simulink model "Simulink_Program_June30_K2andK3"  (R2023b)
settings: Solver=VariableStepAuto  StartTime=0.0  StopTime=1  RelTol=1e-3
libraries: fl_lib x11, nesl_utility x9, ee_lib x7, SignalEditorBlockLib x1
settings Model: Creator=romul  LastModifiedBy=OWNER

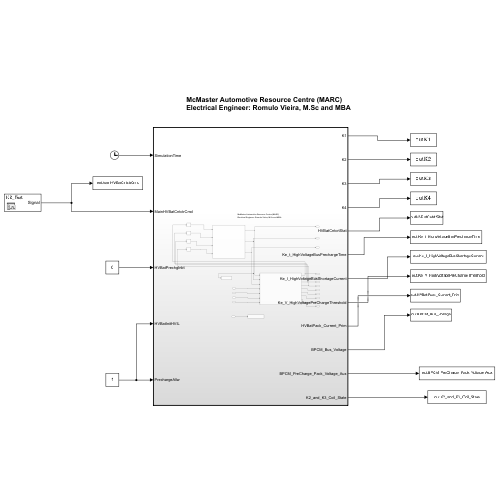
[thumbnail: Simulink's stored preview of the top-level diagram]
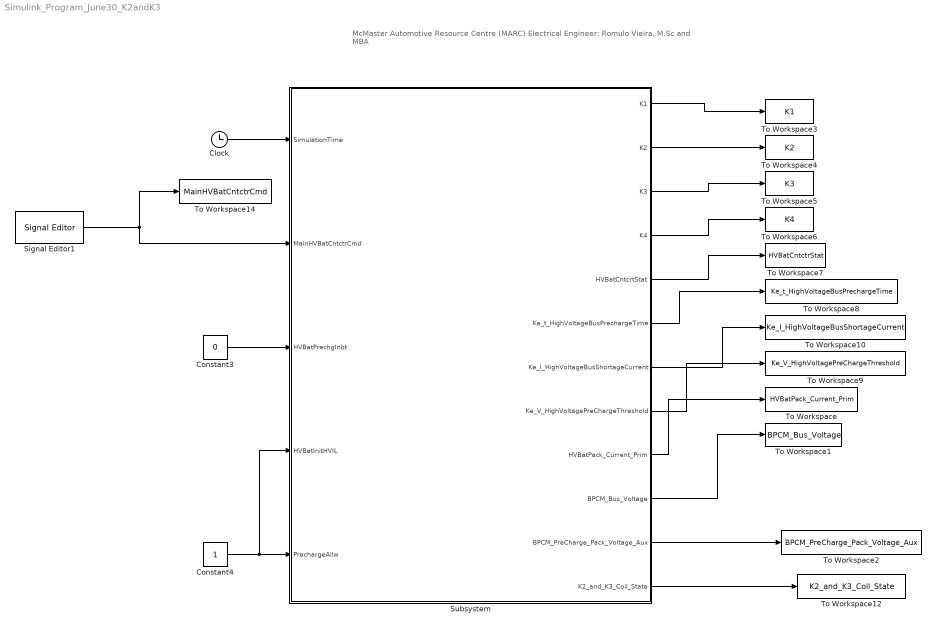
== system Simulink_Program_June30_K2andK3 ==
  note: McMaster Automotive Resource Centre (MARC)
      | Electrical Engineer: Romulo Vieira, M.Sc and MBA
  Clock : Clock
  Constant3 : Constant  Value=0
  Constant4 : Constant
  Signal Editor1 : SignalEditorBlockLib/Signal Editor  FileName=K2_Test.mat  ActiveScenario=K2_Test  ActiveSignal=Signal  IsBus=off  OutputBusObjectStr=Bus: BusObject  SampleTime=0  Interpolate=off  ZeroCross=off  OutputAfterFinalValue=Setting to zero  Unit=inherit  PreserveSignalName=on  ApplySigPropsToAllScenarios=on  ApplySigPropsToAllSignals=off
  Subsystem : Subsystem  TreatAsAtomicUnit=on
  To Workspace : ToWorkspace  VariableName=HVBatPack_Current_Prim  SampleTime=-1
  To Workspace1 : ToWorkspace  VariableName=BPCM_Bus_Voltage  SampleTime=-1
  To Workspace10 : ToWorkspace  VariableName=Ke_I_HighVoltageBusShortageCurrent  SampleTime=-1
  To Workspace12 : ToWorkspace  VariableName=K2_and_K3_Coil_State  SampleTime=-1
  To Workspace14 : ToWorkspace  VariableName=MainHVBatCntctrCmd  SaveFormat=Timeseries  SampleTime=-1
  To Workspace2 : ToWorkspace  VariableName=BPCM_PreCharge_Pack_Voltage_Aux  SampleTime=-1
  To Workspace3 : ToWorkspace  VariableName=K1  SaveFormat=Timeseries  SampleTime=-1
  To Workspace4 : ToWorkspace  VariableName=K2  SaveFormat=Timeseries  SampleTime=-1
  To Workspace5 : ToWorkspace  VariableName=K3  SaveFormat=Timeseries  SampleTime=-1
  To Workspace6 : ToWorkspace  VariableName=K4  SampleTime=-1
  To Workspace7 : ToWorkspace  VariableName=HVBatCntctrStat  SampleTime=-1
  To Workspace8 : ToWorkspace  VariableName=Ke_t_HighVoltageBusPrechargeTime  SampleTime=-1
  To Workspace9 : ToWorkspace  VariableName=Ke_V_HighVoltagePreChargeThreshold  SampleTime=-1
  wires:
  Subsystem/4(K4) -> To Workspace6/1
  Subsystem/12(K2_and_K3_Coil_State) -> To Workspace12/1
  Subsystem/7(Ke_I_HighVoltageBusShortageCurrent) -> To Workspace10/1
  Subsystem/1(K1) -> To Workspace3/1
  Clock/1 -> Subsystem/1(SimulationTime)
  Constant3/1 -> Subsystem/3(HVBatPrechgInbt)
  Subsystem/2(K2) -> To Workspace4/1
  Subsystem/8(Ke_V_HighVoltagePreChargeThreshold) -> To Workspace9/1
  Subsystem/3(K3) -> To Workspace5/1
  Constant4/1 -> Subsystem/5(PrechargeAllw), Subsystem/4(HVBatInitHVIL)
  Subsystem/11(BPCM_PreCharge_Pack_Voltage_Aux) -> To Workspace2/1
  Subsystem/6(Ke_t_HighVoltageBusPrechargeTime) -> To Workspace8/1
  Subsystem/5(HVBatCntcrtStat) -> To Workspace7/1
  Subsystem/10(BPCM_Bus_Voltage) -> To Workspace1/1
  Subsystem/9(HVBatPack_Current_Prim) -> To Workspace/1
  Signal Editor1/1 -> To Workspace14/1, Subsystem/2(MainHVBatCntctrCmd)

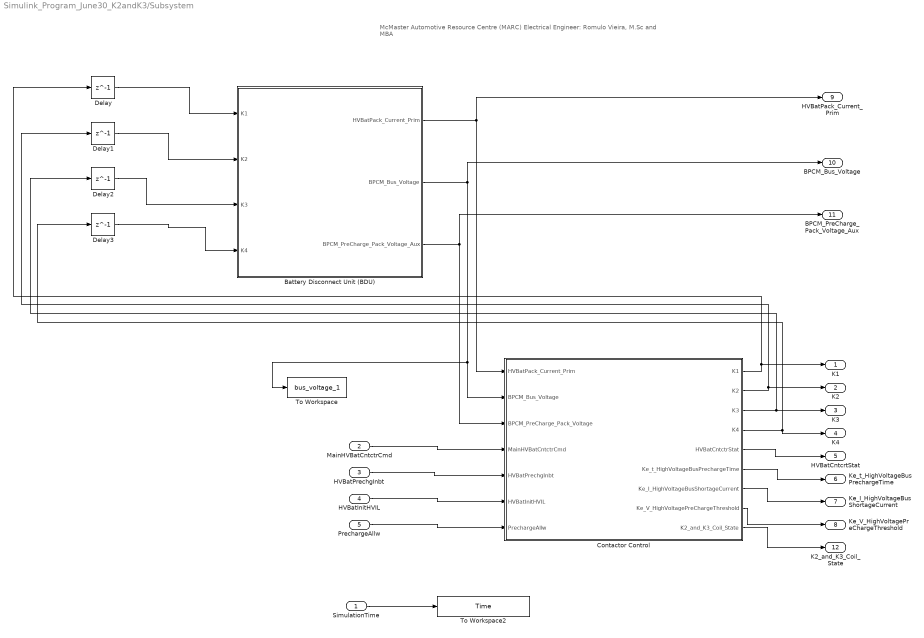
== system Simulink_Program_June30_K2andK3/Subsystem ==
  note: McMaster Automotive Resource Centre (MARC)
      | Electrical Engineer: Romulo Vieira, M.Sc and MBA
  SimulationTime : Inport
  MainHVBatCntctrCmd : Inport  Port=2
  HVBatPrechgInbt : Inport  Port=3
  HVBatInitHVIL : Inport  Port=4
  PrechargeAllw : Inport  Port=5
  Battery Disconnect Unit (BDU) : Subsystem  TreatAsAtomicUnit=on
  Contactor Control : Subsystem  TreatAsAtomicUnit=on
  Delay{,1..3} (4 alike) : Delay  DelayLength=1
  To Workspace : ToWorkspace  VariableName=bus_voltage_1  SaveFormat=Timeseries  SampleTime=-1
  To Workspace2 : ToWorkspace  VariableName=Time  SampleTime=0.001
  K1 : Outport
  K2 : Outport  Port=2
  K3 : Outport  Port=3
  K4 : Outport  Port=4
  HVBatCntcrtStat : Outport  Port=5
  Ke_t_HighVoltageBusPrechargeTime : Outport  Port=6
  Ke_I_HighVoltageBusShortageCurrent : Outport  Port=7
  Ke_V_HighVoltagePreChargeThreshold : Outport  Port=8
  HVBatPack_Current_Prim : Outport  Port=9
  BPCM_Bus_Voltage : Outport  Port=10
  BPCM_PreCharge_Pack_Voltage_Aux : Outport  Port=11
  K2_and_K3_Coil_State : Outport  Port=12
  wires:
  Battery Disconnect Unit (BDU)/1(HVBatPack_Current_Prim) -> HVBatPack_Current_Prim/1, Contactor Control/1(HVBatPack_Current_Prim)
  HVBatPrechgInbt/1 -> Contactor Control/5(HVBatPrechgInbt)
  HVBatInitHVIL/1 -> Contactor Control/6(HVBatInitHVIL)
  PrechargeAllw/1 -> Contactor Control/7(PrechargeAllw)
  Contactor Control/1(K1) -> K1/1, Delay/1
  Contactor Control/2(K2) -> Delay1/1, K2/1
  Contactor Control/3(K3) -> Delay2/1, K3/1
  Contactor Control/4(K4) -> Delay3/1, K4/1
  Contactor Control/5(HVBatCntctrStat) -> HVBatCntcrtStat/1
  Contactor Control/6(Ke_t_HighVoltageBusPrechargeTime) -> Ke_t_HighVoltageBusPrechargeTime/1
  Contactor Control/7(Ke_I_HighVoltageBusShortageCurrent) -> Ke_I_HighVoltageBusShortageCurrent/1
  Contactor Control/8(Ke_V_HighVoltagePreChargeThreshold) -> Ke_V_HighVoltagePreChargeThreshold/1
  Battery Disconnect Unit (BDU)/3(BPCM_PreCharge_Pack_Voltage_Aux) -> BPCM_PreCharge_Pack_Voltage_Aux/1, Contactor Control/3(BPCM_PreCharge_Pack_Voltage)
  Delay/1 -> Battery Disconnect Unit (BDU)/1(K1)
  Delay1/1 -> Battery Disconnect Unit (BDU)/2(K2)
  Delay2/1 -> Battery Disconnect Unit (BDU)/3(K3)
  Delay3/1 -> Battery Disconnect Unit (BDU)/4(K4)
  SimulationTime/1 -> To Workspace2/1
  Battery Disconnect Unit (BDU)/2(BPCM_Bus_Voltage) -> BPCM_Bus_Voltage/1, Contactor Control/2(BPCM_Bus_Voltage), To Workspace/1
  Contactor Control/9(K2_and_K3_Coil_State) -> K2_and_K3_Coil_State/1
  MainHVBatCntctrCmd/1 -> Contactor Control/4(MainHVBatCntctrCmd)

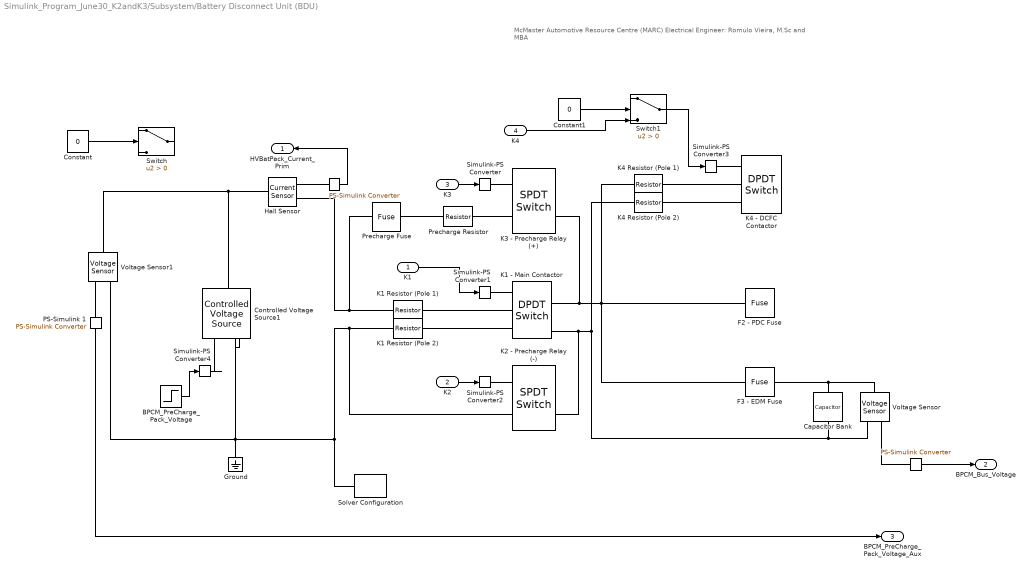
== system Simulink_Program_June30_K2andK3/Subsystem/Battery Disconnect Unit (BDU) ==
  note: McMaster Automotive Resource Centre (MARC)
      | Electrical Engineer: Romulo Vieira, M.Sc and MBA
  K1 : Inport
  K2 : Inport  Port=2
  K3 : Inport  Port=3
  K4 : Inport  Port=4
  "   " : nesl_utility/PS-Simulink Converter  PhysicalDomain=network_engine_domain  SubClassName=ps_output  LeftPortType=input  RightPortType=output  PseudoPeriodic=off  Frequencies=[]  VectorFormat=inherit  Unit=inherit  AffineConversion=off
  " " : nesl_utility/PS-Simulink Converter  PhysicalDomain=network_engine_domain  SubClassName=ps_output  LeftPortType=input  RightPortType=output  PseudoPeriodic=off  Frequencies=[]  VectorFormat=inherit  Unit=inherit  AffineConversion=off
  BPCM_PreCharge_Pack_Voltage : Step  Time=0  After=450  SampleTime=0.001
  Capacitor Bank : fl_lib/Electrical/Electrical Elements/Capacitor  c=750e-6 F  r=1e-6 Ohm  g=0 1/Ohm  i_specify=off  i_priority=None  i=0 A  i_nominal_specify=off  i_nominal_unit=A  i_nominal_value=1  v_specify=off  v_priority=None  v=0 V  v_nominal_specify=off  v_nominal_unit=V  v_nominal_value=1  vc_specify=on  vc_priority=High  vc=0 V  vc_nominal_specify=off  vc_nominal_unit=V  vc_nominal_value=1
  Constant : Constant  Value=0
  Constant1 : Constant  Value=0
  Controlled Voltage Source1 : fl_lib/Electrical/Electrical Sources/Controlled Voltage Source
  F2 - PDC Fuse : ee_lib/Switches & Breakers/Fuse  prm=1  I_rated=125 A  melt_margin=1  T_fuse=0 s  I2t=1 A^2*s  I_vec=[1.9, 2, 2.5, 30] A  t_vec=[10000, 1, .3, .001] s  R_closed=0.01 Ohm  G_open=1e-8 1/Ohm  exposemeasurement=ee.enum.exposemeasurement.hidden
      settings: InternalSimscapePortConfiguration="{\"Bottom\":[],\"Left\":[{\"id\":\"p\",\"label\":\"\",\"type\":\"foundation.electrical.electrical\"}],\"Right\":[{\"id\":\"n\",\"label\":\"\",\"type\":\"foundation.electrical.electrical\"}],\"Top\":[]}"
  F3 - EDM Fuse : ee_lib/Switches & Breakers/Fuse  prm=1  I_rated=600 A  melt_margin=1  T_fuse=0 s  I2t=1 A^2*s  I_vec=[1.9, 2, 2.5, 30] A  t_vec=[10000, 1, .3, .001] s  R_closed=0.01 Ohm  G_open=1e-8 1/Ohm  exposemeasurement=ee.enum.exposemeasurement.hidden
      settings: InternalSimscapePortConfiguration="{\"Bottom\":[],\"Left\":[{\"id\":\"p\",\"label\":\"\",\"type\":\"foundation.electrical.electrical\"}],\"Right\":[{\"id\":\"n\",\"label\":\"\",\"type\":\"foundation.electrical.electrical\"}],\"Top\":[]}"
  Ground : fl_lib/Electrical/Electrical Elements/Electrical Reference
  Hall Sensor : fl_lib/Electrical/Electrical Sensors/Current Sensor
  K1 - Main Contactor : ee_lib/Switches & Breakers/DPDT Switch  R_closed=0.01 Ohm  G_open=1e-6 S  Threshold=0.5 V  Width=0 V  model_dynamics=0  t_on=1e-3 s  t_off=1e-3 s  initial_vT=0 V
      settings: InternalSimscapePortConfiguration="{\"Bottom\":[],\"Left\":[{\"id\":\"vT\",\"label\":\"vT\",\"type\":\"input\"},{\"id\":\"p1\",\"label\":\"\",\"type\":\"foundation.electrical.electrical\"},{\"id\":\"p2\",\"label\":\"\",\"type\":\"foundation.electrical.electrical\"}],\"Right\":[{\"id\":\"n11\",\"label\":\"\",\"type\":\"foundation.electrical.electrical\"},{\"id\":\"n12\",\"label\":\"\",\"type\":\"foundation.electrical.electrical\"},{\"id\":\"n21\",\"label\":\"\",\"type\":\"foundation.electrical.electrical\"},{\"id\":\"n22\",\"label\":\"\",\"type\":\"foundation.electrical.electrical\"}],\"Top\":[]}"
  K1 Resistor (Pole 1) : fl_lib/Electrical/Electrical Elements/Resistor  R=0.0003 Ohm  i_specify=off  i_priority=None  i=0 A  i_nominal_specify=off  i_nominal_unit=A  i_nominal_value=1  v_specify=off  v_priority=None  v=0 V  v_nominal_specify=off  v_nominal_unit=V  v_nominal_value=1
  K1 Resistor (Pole 2) : fl_lib/Electrical/Electrical Elements/Resistor  R=0.0003 Ohm  i_specify=off  i_priority=None  i=0 A  i_nominal_specify=off  i_nominal_unit=A  i_nominal_value=1  v_specify=off  v_priority=None  v=0 V  v_nominal_specify=off  v_nominal_unit=V  v_nominal_value=1
  K2 - Precharge Relay (-) : ee_lib/Switches & Breakers/SPDT Switch  R_closed=0.01 Ohm  G_open=1e-6 S  Threshold=0.5 V  Width=0 V  model_dynamics=0  t_on=1e-3 s  t_off=1e-3 s  initial_vT=0 V
  K3 - Precharge Relay (+) : ee_lib/Switches & Breakers/SPDT Switch  R_closed=0.01 Ohm  G_open=1e-6 S  Threshold=0.5 V  Width=0 V  model_dynamics=0  t_on=1e-3 s  t_off=1e-3 s  initial_vT=0 V
  K4 - DCFC Contactor : ee_lib/Switches & Breakers/DPDT Switch  R_closed=0.01 Ohm  G_open=1e-6 S  Threshold=0.5 V  Width=0 V  model_dynamics=0  t_on=1e-3 s  t_off=1e-3 s  initial_vT=0 V
      settings: InternalSimscapePortConfiguration="{\"Bottom\":[],\"Left\":[{\"id\":\"vT\",\"label\":\"vT\",\"type\":\"input\"},{\"id\":\"p1\",\"label\":\"\",\"type\":\"foundation.electrical.electrical\"},{\"id\":\"p2\",\"label\":\"\",\"type\":\"foundation.electrical.electrical\"}],\"Right\":[{\"id\":\"n11\",\"label\":\"\",\"type\":\"foundation.electrical.electrical\"},{\"id\":\"n12\",\"label\":\"\",\"type\":\"foundation.electrical.electrical\"},{\"id\":\"n21\",\"label\":\"\",\"type\":\"foundation.electrical.electrical\"},{\"id\":\"n22\",\"label\":\"\",\"type\":\"foundation.electrical.electrical\"}],\"Top\":[]}"
  K4 Resistor (Pole 1) : fl_lib/Electrical/Electrical Elements/Resistor  R=0.0003 Ohm  i_specify=off  i_priority=None  i=0 A  i_nominal_specify=off  i_nominal_unit=A  i_nominal_value=1  v_specify=off  v_priority=None  v=0 V  v_nominal_specify=off  v_nominal_unit=V  v_nominal_value=1
  K4 Resistor (Pole 2) : fl_lib/Electrical/Electrical Elements/Resistor  R=0.0003 Ohm  i_specify=off  i_priority=None  i=0 A  i_nominal_specify=off  i_nominal_unit=A  i_nominal_value=1  v_specify=off  v_priority=None  v=0 V  v_nominal_specify=off  v_nominal_unit=V  v_nominal_value=1
  PS-Simulink 1 : nesl_utility/PS-Simulink Converter  PhysicalDomain=network_engine_domain  SubClassName=ps_output  LeftPortType=input  RightPortType=output  PseudoPeriodic=off  Frequencies=[]  VectorFormat=inherit  Unit=inherit  AffineConversion=off
  Precharge Fuse : ee_lib/Switches & Breakers/Fuse  prm=1  I_rated=600 A  melt_margin=1  T_fuse=0 s  I2t=1 A^2*s  I_vec=[1.9, 2, 2.5, 30] A  t_vec=[10000, 1, .3, .001] s  R_closed=0.01 Ohm  G_open=1e-8 1/Ohm  exposemeasurement=ee.enum.exposemeasurement.hidden
      settings: InternalSimscapePortConfiguration="{\"Bottom\":[],\"Left\":[{\"id\":\"p\",\"label\":\"\",\"type\":\"foundation.electrical.electrical\"}],\"Right\":[{\"id\":\"n\",\"label\":\"\",\"type\":\"foundation.electrical.electrical\"}],\"Top\":[]}"
  Precharge Resistor : fl_lib/Electrical/Electrical Elements/Resistor  R=25 Ohm  i_specify=off  i_priority=None  i=0 A  i_nominal_specify=off  i_nominal_unit=A  i_nominal_value=1  v_specify=off  v_priority=None  v=0 V  v_nominal_specify=off  v_nominal_unit=V  v_nominal_value=1
  Simulink-PS Converter{,1..3} (4 alike) : nesl_utility/Simulink-PS Converter  PhysicalDomain=network_engine_domain  SubClassName=ps_input  LeftPortType=input  RightPortType=output  PseudoPeriodic=off  Frequencies=[]  NoiseDistribution=none  NoiseParameters=[]  Unit=1  AffineConversion=off  FilteringAndDerivatives=provide  SimscapeFilterOrder=1  InputFilterTimeConstant=0.001  UdotUserProvided=0
  Simulink-PS Converter4 : nesl_utility/Simulink-PS Converter  PhysicalDomain=network_engine_domain  SubClassName=ps_input  LeftPortType=input  RightPortType=output  PseudoPeriodic=off  Frequencies=[]  NoiseDistribution=none  NoiseParameters=[]  Unit=1  AffineConversion=off  FilteringAndDerivatives=filter  SimscapeFilterOrder=1  InputFilterTimeConstant=0.0000001  UdotUserProvided=0
  Solver Configuration : nesl_utility/Solver Configuration  PhysicalDomain=network_engine_domain  SubClassName=solver  LeftPortType=input  RightPortType=generic  Tones=[]  Harmonics=[]  SimulateNoise=off  Profile=off  UseLocalSampling=off  EnableSwitchedLinearOptims=on  FrequencyDomain=off  UseCCode=off  RelTol=0.001  AbsTol=0.001  MinStep=1e-09  ToWorkspace=off  RevertToSquareIcSolve=off  NumHomotopyIterations=100  PhasorMode=off  PhasorModeNumHarmonics=1  ConsistencySolver=NEWTON_XTOL_AFTER_FTOL  IndexReductionMethod=DerivativeReplacement  DoDC=off  ResidualTolerance=1e-09  ConsistencyTolSource=GLOBAL  ConsistencyAbsTol=0.001  ConsistencyRelTol=0.001  ConsistencyTolFactor=0.001  UseLocalSolver=off  LocalSolverChoice=NE_BACKWARD_EULER_ADVANCER  ResolveIndetEquations=on  FunctionEvalNumThread=1  LocalSolverSampleTime=0.001  DoFixedCost=off  MaxNonlinIter=3  MaxModeIter=2  ComputeImpulses=off  ImpulseIterations=2  LinearAlgebra=auto  LinearAlgebraNumThread=0  EquationFormulation=NE_TIME_EF  DelaysMemoryBudget=1024  AutomaticFiltering=on  FilteringTimeConstant=0.001  PartitionStorageMethod=AS_NEEDED  PartitionMemoryBudget=1024  PartitionMethod=ROBUST  MultibodyUseLocalSolver=off  MultibodyLocalSolverChoice=ODE1  MultibodyLocalSolverSampleTime=0.001
  Switch : Switch  Criteria=u2 > Threshold  SaturateOnIntegerOverflow=off  InputSameDT=off
  Switch1 : Switch  Criteria=u2 > Threshold  SaturateOnIntegerOverflow=off  InputSameDT=off
  Voltage Sensor : fl_lib/Electrical/Electrical Sensors/Voltage Sensor
  Voltage Sensor1 : fl_lib/Electrical/Electrical Sensors/Voltage Sensor
  HVBatPack_Current_Prim : Outport
  BPCM_Bus_Voltage : Outport  Port=2
  BPCM_PreCharge_Pack_Voltage_Aux : Outport  Port=3
  wires:
  Switch1/1 -> Simulink-PS Converter3/1
  K3/1 -> Simulink-PS Converter/1
  "   "/1 -> HVBatPack_Current_Prim/1
  K2/1 -> Simulink-PS Converter2/1
  BPCM_PreCharge_Pack_Voltage/1 -> Simulink-PS Converter4/1
  PS-Simulink 1/1 -> BPCM_PreCharge_Pack_Voltage_Aux/1
  " "/1 -> BPCM_Bus_Voltage/1
  K1/1 -> Simulink-PS Converter1/1
  Constant1/1 -> Switch1/2
  K4/1 -> Switch1/3
  ? -> Switch1/1
  ? -> Switch/1
  ? -> Switch/3
  Constant/1 -> Switch/2
  connections:
  K1 Resistor (Pole 2)/LConn1 -- K1 - Main Contactor/LConn3
  Capacitor Bank/LConn1 -- Voltage Sensor/LConn1 -- F3 - EDM Fuse/LConn1
  K2 - Precharge Relay (-)/RConn2 -- K1 - Main Contactor/RConn4 -- Voltage Sensor/RConn2 -- Capacitor Bank/RConn1 -- K4 Resistor (Pole 2)/RConn1
  Hall Sensor/RConn2 -- Precharge Fuse/LConn1 -- K1 Resistor (Pole 1)/RConn1
  K3 - Precharge Relay (+)/RConn2 -- K4 Resistor (Pole 1)/RConn1 -- F2 - PDC Fuse/RConn1 -- F3 - EDM Fuse/RConn1 -- K1 - Main Contactor/RConn2
  Precharge Resistor/LConn1 -- K3 - Precharge Relay (+)/LConn2
  Simulink-PS Converter2/RConn1 -- K2 - Precharge Relay (-)/LConn1
  Precharge Resistor/RConn1 -- Precharge Fuse/RConn1
  Simulink-PS Converter1/RConn1 -- K1 - Main Contactor/LConn1
  Controlled Voltage Source1/LConn1 -- Hall Sensor/LConn1 -- Voltage Sensor1/LConn1
  Simulink-PS Converter/RConn1 -- K3 - Precharge Relay (+)/LConn1
  Voltage Sensor/RConn1 -- " "/LConn1
  K4 - DCFC Contactor/LConn1 -- Simulink-PS Converter3/RConn1
  "   "/LConn1 -- Hall Sensor/RConn1
  Simulink-PS Converter4/RConn1 -- Controlled Voltage Source1/RConn1
  Voltage Sensor1/RConn1 -- PS-Simulink 1/LConn1
  K1 Resistor (Pole 1)/LConn1 -- K1 - Main Contactor/LConn2
  Solver Configuration/RConn1 -- Ground/LConn1 -- Voltage Sensor1/RConn2 -- Controlled Voltage Source1/RConn2 -- K2 - Precharge Relay (-)/LConn2 -- K1 Resistor (Pole 2)/RConn1
  K4 - DCFC Contactor/LConn2 -- K4 Resistor (Pole 1)/LConn1
  K4 Resistor (Pole 2)/LConn1 -- K4 - DCFC Contactor/LConn3

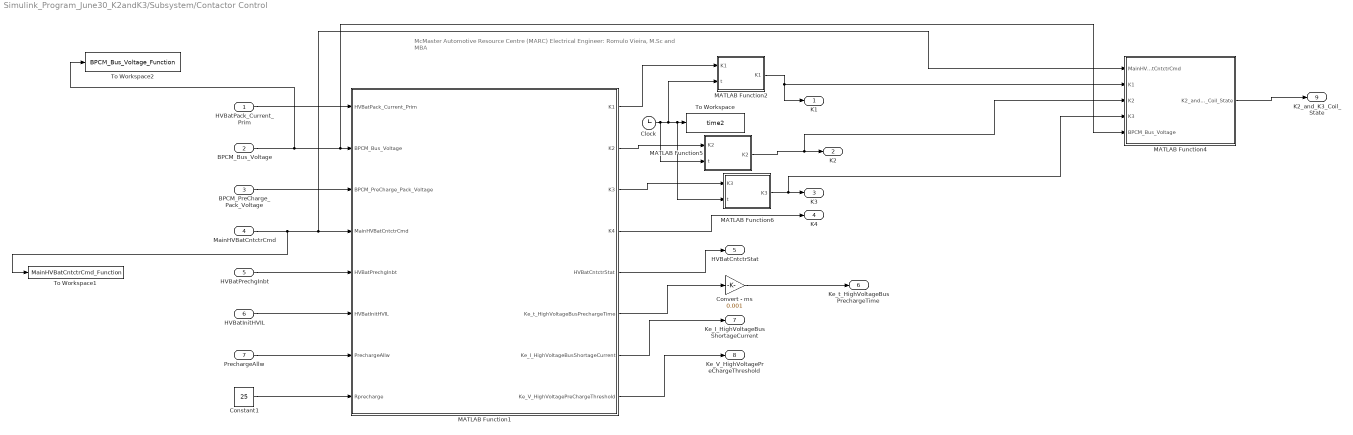
== system Simulink_Program_June30_K2andK3/Subsystem/Contactor Control ==
  note: McMaster Automotive Resource Centre (MARC)
      | Electrical Engineer: Romulo Vieira, M.Sc and MBA
  HVBatPack_Current_Prim : Inport
  BPCM_Bus_Voltage : Inport  Port=2
  BPCM_PreCharge_Pack_Voltage : Inport  Port=3
  MainHVBatCntctrCmd : Inport  Port=4
  HVBatPrechgInbt : Inport  Port=5
  HVBatInitHVIL : Inport  Port=6
  PrechargeAllw : Inport  Port=7
  Clock : Clock
  Constant1 : Constant  Value=25
  Convert - ms : Gain  Gain=0.001
  MATLAB Function1 : MATLAB Function  SystemSampleTime=0.001
  MATLAB Function2 : MATLAB Function  TreatAsAtomicUnit=on
  MATLAB Function4 : MATLAB Function  TreatAsAtomicUnit=on
  MATLAB Function5 : MATLAB Function  TreatAsAtomicUnit=on
  MATLAB Function6 : MATLAB Function  TreatAsAtomicUnit=on
  To Workspace : ToWorkspace  VariableName=time2  SampleTime=-1
  To Workspace1 : ToWorkspace  VariableName=MainHVBatCntctrCmd_Function  SaveFormat=Timeseries  SampleTime=-1
  To Workspace2 : ToWorkspace  VariableName=BPCM_Bus_Voltage_Function  SaveFormat=Timeseries  SampleTime=-1
  K1 : Outport
  K2 : Outport  Port=2
  K3 : Outport  Port=3
  K4 : Outport  Port=4
  HVBatCntctrStat : Outport  Port=5
  Ke_t_HighVoltageBusPrechargeTime : Outport  Port=6
  Ke_I_HighVoltageBusShortageCurrent : Outport  Port=7
  Ke_V_HighVoltagePreChargeThreshold : Outport  Port=8
  K2_and_K3_Coil_State : Outport  Port=9
  wires:
  HVBatPack_Current_Prim/1 -> MATLAB Function1/1(HVBatPack_Current_Prim)
  PrechargeAllw/1 -> MATLAB Function1/7(PrechargeAllw)
  BPCM_PreCharge_Pack_Voltage/1 -> MATLAB Function1/3(BPCM_PreCharge_Pack_Voltage)
  Constant1/1 -> MATLAB Function1/8(Rprecharge)
  MATLAB Function1/7(Ke_I_HighVoltageBusShortageCurrent) -> Ke_I_HighVoltageBusShortageCurrent/1
  HVBatInitHVIL/1 -> MATLAB Function1/6(HVBatInitHVIL)
  HVBatPrechgInbt/1 -> MATLAB Function1/5(HVBatPrechgInbt)
  MATLAB Function1/5(HVBatCntctrStat) -> HVBatCntctrStat/1
  MATLAB Function1/6(Ke_t_HighVoltageBusPrechargeTime) -> Convert - ms/1
  MATLAB Function1/8(Ke_V_HighVoltagePreChargeThreshold) -> Ke_V_HighVoltagePreChargeThreshold/1
  Convert - ms/1 -> Ke_t_HighVoltageBusPrechargeTime/1
  MATLAB Function4/1(K2_and_K3_Coil_State) -> K2_and_K3_Coil_State/1
  MATLAB Function1/4(K4) -> K4/1
  Clock/1 -> MATLAB Function5/2(t), MATLAB Function2/2(t), MATLAB Function6/2(t), To Workspace/1
  BPCM_Bus_Voltage/1 -> MATLAB Function4/5(BPCM_Bus_Voltage), MATLAB Function1/2(BPCM_Bus_Voltage), To Workspace2/1
  MainHVBatCntctrCmd/1 -> To Workspace1/1, MATLAB Function4/1(MainHVBatCntctrCmd), MATLAB Function1/4(MainHVBatCntctrCmd)
  MATLAB Function1/2(K2) -> MATLAB Function5/1("K2 ")
  MATLAB Function5/1(K2) -> MATLAB Function4/3(K2), K2/1
  MATLAB Function1/3(K3) -> MATLAB Function6/1("K3 ")
  MATLAB Function6/1(K3) -> MATLAB Function4/4(K3), K3/1
  MATLAB Function1/1(K1) -> MATLAB Function2/1("K1 ")
  MATLAB Function2/1(K1) -> MATLAB Function4/2(K1), K1/1

== matlab function Simulink_Program_June30_K2andK3/Subsystem/Contactor Control/MATLAB Function1 ==
  settings: updateMethod=DISCRETE
  data: HVBatPack_Current_Prim input; BPCM_Bus_Voltage input; BPCM_PreCharge_Pack_Voltage input; MainHVBatCntctrCmd input; K1 output; HVBatPrechgInbt input; HVBatInitHVIL input; PrechargeAllw input; K2 output; K3 output; K4 output; HVBatCntctrStat output; Ke_t_HighVoltageBusPrechargeTime output; Ke_I_HighVoltageBusShortageCurrent output; Ke_V_HighVoltagePreChargeThreshold output; Rprecharge input
% McMaster Automotive Resource Centre (MARC)
% Electrical Engineer: Romulo Vieira, M.Sc and MBA - PhD Candidate
function [K1, K2, K3, K4, HVBatCntctrStat, Ke_t_HighVoltageBusPrechargeTime, Ke_I_HighVoltageBusShortageCurrent, Ke_V_HighVoltagePreChargeThreshold] = prechargeSequencerNoClock( ...
     HVBatPack_Current_Prim, BPCM_Bus_Voltage, BPCM_PreCharge_Pack_Voltage, MainHVBatCntctrCmd, HVBatPrechgInbt, HVBatInitHVIL, PrechargeAllw, Rprecharge)

%-----------------------------------------------------------
% Purpose: Manage precharge relay and contactor sequence without an external clock
% Controls how the HV bus charges up safely to near pack voltage
% Tracks time window where precharge relays were active
%-----------------------------------------------------------

% Declare persistent variables (retain values across function calls)
persistent I_buffer V_buffer idx Stage HVBatCntctrStat_Aux Ke_idx fill_count last_PrechargeAllw stage2_count TimeSincePrechargeStart

% Declare constants
Buffer_length                      = 100; % Buffer to store 100 ms worth of data (1 ms sample rate in Matlab function)
Ke_V_HighVoltagePreChargeThreshold = 0.99 * BPCM_PreCharge_Pack_Voltage; % Target voltage: 98.5% of pack voltage
Unset_Ke_idx                       = -1; % Marker to indicate target not reached yet
Min_Stage2_Samples                 = 1; % Minimum time (samples) to stay in Stage 2

% Initialize persistent variables on first call
if isempty(I_buffer)
    I_buffer            = zeros(Buffer_length,1); % Precharge current buffer
    V_buffer            = zeros(Buffer_length,1); % Precharge voltage buffer
    idx                 = 1; % Index for buffers
    Stage               = 0; % Initial internal stage
    HVBatCntctrStat_Aux = 0; % Initial stage for the contactor control
    Ke_idx              = Unset_Ke_idx; % Target voltage not reached yet
    fill_count          = 0; % Counter for Stage 1 samples
    last_PrechargeAllw  = 0; % Track previous PrechargeAllw
    stage2_count        = 0; % Counter for Stage 2 duration
end

if isempty(TimeSincePrechargeStart)
    TimeSincePrechargeStart = 0;
end

% Default outputs
K1 = 0; K2 = 0; K3 = 0; K4 = 0;
HVBatCntctrStat = HVBatCntctrStat_Aux;

switch Stage
    case 0
        % All contactors off
        if MainHVBatCntctrCmd == 1 && HVBatPrechgInbt == 0 && HVBatInitHVIL == 1 && PrechargeAllw == 1
            % Start precharge
            Stage = 1;
            HVBatCntctrStat_Aux = 1;
            I_buffer(:) = 0;
            V_buffer(:) = 0;
            idx = 1;
            Ke_idx = Unset_Ke_idx;
            fill_count = 0;
            stage2_count = 0;
        end

    case 1
        % Precharge relays on
        K1 = 0; K2 = 1; K3 = 1; K4 = 0;

        if fill_count == 0
            % First precharge sample: log initial current from Vpack and V_HVbus = 0
            I_buffer(idx) = BPCM_PreCharge_Pack_Voltage / Rprecharge; % expected initial current at t=0
        else
            % Normal logging
            I_buffer(idx) = HVBatPack_Current_Prim;
        end
        V_buffer(idx) = BPCM_Bus_Voltage;

        % Check if Vtarget first hit
        if Ke_idx == Unset_Ke_idx && BPCM_Bus_Voltage >= Ke_V_HighVoltagePreChargeThreshold
            Ke_idx = fill_count + 1; % Save when Vtarget was first hit
        end

        % Update fill count
        fill_count = fill_count + 1;

        % Increment and wrap index
        idx = idx + 1;
        if idx > Buffer_length
            idx = 1;
        end

        % Evaluate conditions
        maxI = max(I_buffer);

        if Ke_idx ~= Unset_Ke_idx
            delta_samples = Ke_idx;
        else
            delta_samples = fill_count; % in progress
        end

        if Ke_idx ~= Unset_Ke_idx && delta_samples <= Buffer_length && maxI > 10
            % Success → move to Stage 2
            Stage = 2;
            HVBatCntctrStat_Aux = 1;
            stage2_count = 0; % Start counting Stage 2 duration
        elseif fill_count >= Buffer_length
            Stage = 0; % Fail: reset
            HVBatCntctrStat_Aux = 0;
        end

    case 2
        % Main contactor on, precharge relays also on
        K1 = 1; K2 = 0; K3 = 0; K4 = 0;

        % Increment Stage 2 counter
        stage2_count = stage2_count + 1;

        % Check if we've stayed long enough
        if stage2_count >= Min_Stage2_Samples
            Stage = 3;
            HVBatCntctrStat_Aux = 2;
        end

        if MainHVBatCntctrCmd == 0
            % VCU revoked main command unexpectedly
            Stage = 0;
            HVBatCntctrStat_Aux = 4;  % PreCharge_Inhibited or equivalent
        end
        
        if K1 == 0
            % Main contactor unexpectedly opened
            Stage = 0;
            HVBatCntctrStat_Aux = 3;  % PreCharge_Failed or similar
        end

    case 3
        % Stay latched in Stage 3 until PrechargeAllw 0->1 transition
        K1 = 1; K2 = 0; K3 = 0; K4 = 0;

        if last_PrechargeAllw == 0 && PrechargeAllw == 1
            % Detected re-arm condition
            Stage = 0;
            HVBatCntctrStat_Aux = 0;
            I_buffer(:) = 0;
            V_buffer(:) = 0;
            idx = 1;
            Ke_idx = Unset_Ke_idx;
            fill_count = 0;
            stage2_count = 0;
        end

    otherwise
        % Safety fallback
        K1 = 0; K2 = 0; K3 = 0; K4 = 0;
        Stage = 0;
        HVBatCntctrStat_Aux = 0;
end

HVBatCntctrStat = HVBatCntctrStat_Aux;

% Debug outputs
Ke_t_HighVoltageBusPrechargeTime = Ke_idx;
Ke_I_HighVoltageBusShortageCurrent = max(I_buffer);

if Ke_t_HighVoltageBusPrechargeTime < 0
    Ke_t_HighVoltageBusPrechargeTime = 0;
else
    Ke_t_HighVoltageBusPrechargeTime = Ke_t_HighVoltageBusPrechargeTime + Min_Stage2_Samples;
end

% Update last_PrechargeAllw for edge detection
last_PrechargeAllw = PrechargeAllw;

% K1 Coil State Diagnostic (Enumerated as integers)
% 0 = OPEN
% 1 = CLOSED
% 2 = SHORTED_HIGH
% 3 = SHORTED_LOW
% 4 = NORMAL

% if K2 == 1 && K3 == 1
%     TimeSincePrechargeStart = TimeSincePrechargeStart + 1;
% else 
%     TimeSincePrechargeStart = 0;
% end
% 
% % if MainHVBatCntctrCmd == 0 && BPCM_Bus_Voltage > 270
% %     K1_Coil_State = 3; % SHORTED_HIGH
% % elseif MainHVBatCntctrCmd == 1 && BPCM_Bus_Voltage <= 270 && TimeSincePrechargeStart > 90
% %     K1_Coil_State = 4; % SHORTED_LOW
% % elseif MainHVBatCntctrCmd == 1 && K1 == 1 && BPCM_Bus_Voltage > 270
% %     K1_Coil_State = 1; % CLOSED
% % elseif (MainHVBatCntctrCmd == 0 && K1 == 0 && BPCM_Bus_Voltage <= 270) || (MainHVBatCntctrCmd == 1 && K1 == 0 && TimeSincePrechargeStart <= 90)
% %     K1_Coil_State = 0; % OPEN
% 
% 
% %% K1 logic
% 
% if MainHVBatCntctrCmd == 0 && K1 == 0 && BPCM_Bus_Voltage <= 270
%     K1_Coil_State = 0; % OPEN (safe)
% 
% 
% elseif K1 == 0 && BPCM_Bus_Voltage > 270 && (Stage == 2 || Stage == 3)
%     K1_Coil_State = 2; % SHORTED_HIGH (unexpected high voltage without K1)
% 
% elseif MainHVBatCntctrCmd == 0 && K1 == 1
%     K1_Coil_State = 3; % SHORTED_LOW (K1 shouldn't be closed when VCU off)
% 
% 
% elseif MainHVBatCntctrCmd == 1 && K1 == 0 && TimeSincePrechargeStart <= 90
%     K1_Coil_State = 0; % OPEN (precharge in progress)
% 
% 
% elseif MainHVBatCntctrCmd == 1 && K1 == 0 && BPCM_Bus_Voltage <= 270 && TimeSincePrechargeStart > 90
%     K1_Coil_State = 3; % SHORTED_LOW (precharge failed)
% 
% 
% 
% elseif MainHVBatCntctrCmd == 1 && K1 == 1 && BPCM_Bus_Voltage > 270
%     K1_Coil_State = 1; % CLOSED (healthy)
% 
% elseif MainHVBatCntctrCmd == 1 && K1 == 1 && BPCM_Bus_Voltage <= 270
%     K1_Coil_State = 3; % SHORTED_LOW (K1 closed, but no voltage buildup)
% 
% else
%     K1_Coil_State = -1; % Undefined / fallback
% end

% if (MainHVBatCntctrCmd == 0 && K1 == 0 && BPCM_Bus_Voltage <= 270) || (MainHVBatCntctrCmd == 1 && K1 == 0 && TimeSincePrechargeStart <= 90) || ...
%        (MainHVBatCntctrCmd == 1 && K1 == 1 && BPCM_Bus_Voltage > 270)
%     K1_Coil_State = 2; % NORMAL
% end





%% K2 and K3 logic
% if (K2 == 0 && K3 == 0 && BPCM_Bus_Voltage <= 270) || (K2 == 0 && K3 == 0 && K1 == 1)
%     K2_and_K3_Coil_State = 0; % OPEN (idle)
% 
% elseif K2 == 1 && K3 == 1 && BPCM_Bus_Voltage > 0 && TimeSincePrechargeStart <= 90
%     K2_and_K3_Coil_State = 1; % CLOSED (charging)
% 
% elseif K2 == 0 && K3 == 0 && BPCM_Bus_Voltage > 270 && K1 ~= 1
%     K2_and_K3_Coil_State = 2; % SHORTED_HIGH (unexpected voltage without relays)
% 
% elseif K2 == 1 && K3 == 1 && BPCM_Bus_Voltage <= 270 && TimeSincePrechargeStart > 90
%     K2_and_K3_Coil_State = 3; % SHORTED_LOW (relays on but no charge success)
% 
% else
%     K2_and_K3_Coil_State = -1; % Undefined / fallback
% end

% if ((K2 == 0 && K3 == 0 && BPCM_Bus_Voltage <= 270) || (K2 == 1 && K3 == 1 && TimeSincePrechargeStart > 90 && BPCM_Bus_Voltage <= 270)) || (K2 == 1 && K3 == 1 && BPCM_Bus_Voltage > 270 && TimeSincePrechargeStart <= 90)
%     K2_and_K3_Coil_State = 2; % NORMAL
% end




%% K4 logic
% if K1_Coil_State ~= 1
%     % If main contactor not closed, DCFC coil state cannot be trusted or is invalid
%     K4_Coil_State = -1; % Undefined / invalid due to main contactor state
% else
%     % Main contactor is normal, now check DCFC (K4) coil states:
%     if K4 == 0 && BPCM_Bus_Voltage <= 270
%         K4_Coil_State = 0; % OPEN
% 
%     elseif K4 == 1 && BPCM_Bus_Voltage > 270
%         K4_Coil_State = 1; % CLOSED
% 
%     elseif K4 == 0 && BPCM_Bus_Voltage > 270
%         K4_Coil_State = 2; % SHORTED_HIGH
% 
%     elseif K4 == 1 && BPCM_Bus_Voltage <= 270
%         K4_Coil_State = 3; % SHORTED_LOW
% 
%     else
%         K4_Coil_State = -1; % Undefined / fallback
%     end
% 
%     % if (K4 == 0 && BPCM_Bus_Voltage <= 270) || (K4 == 1 && BPCM_Bus_Voltage > 270)
%     %     K4_Coil_State = 2; % NORMAL
%     % end
% end

end

== matlab function Simulink_Program_June30_K2andK3/Subsystem/Contactor Control/MATLAB Function2 ==
  data: K1 input; K1 output; t input
function K1 = fcn(K1, t)
    if t < 0.25 && t >= 0
        if K1 == 1
            K1 = 0;
        end

    elseif  t >= 0.25 && t < 0.34
        if K1 == 1
            K1 = 0;
        end

    elseif t >= 0.34 && t < 0.75 
        if K1 == 1 
            K1 = 0;
        end

    else
        if K1 == 1
            K1 = 0;
        end
    end
end

== matlab function Simulink_Program_June30_K2andK3/Subsystem/Contactor Control/MATLAB Function4 ==
  settings: updateMethod=DISCRETE
  data: MainHVBatCntctrCmd input; K2_and_K3_Coil_State output; K1 input; K2 input; K3 input; BPCM_Bus_Voltage input
function K2_and_K3_Coil_State = fcn(MainHVBatCntctrCmd, K1, K2, K3, BPCM_Bus_Voltage)
% Individual inputs from Simulink Inports

persistent TimeSincePrechargeStart
if isempty(TimeSincePrechargeStart)
    TimeSincePrechargeStart = 0;
end

% Update TimeSincePrechargeStart
if K2 == 1 && K3 == 1
    TimeSincePrechargeStart = TimeSincePrechargeStart + 1;
else
    TimeSincePrechargeStart = 0;
end

% Default state
K2_and_K3_Coil_State = -1;

%% K2 and K3 logic
if (MainHVBatCntctrCmd == 0) || ((K2 == 0 && K3 == 0) && (BPCM_Bus_Voltage <= 270 || K1 == 1))
    K2_and_K3_Coil_State = 0; % OPEN (idle/safe)

elseif K2 == 1 && K3 == 1 && BPCM_Bus_Voltage > 0 && TimeSincePrechargeStart <= 90
    K2_and_K3_Coil_State = 1; % CLOSED (charging)

elseif K2 == 0 && K3 == 0 && BPCM_Bus_Voltage > 270 && K1 ~= 1
    K2_and_K3_Coil_State = 2; % SHORTED_HIGH (unexpected voltage without relays)

elseif K2 == 1 && K3 == 1 && BPCM_Bus_Voltage <= 270 && TimeSincePrechargeStart > 90
    K2_and_K3_Coil_State = 3; % SHORTED_LOW (Relays active too long with no voltage rise)

elseif K2 == 1 && K3 == 1 && K1 ~= 1 && TimeSincePrechargeStart > 90
    K2_and_K3_Coil_State = 3; % SHORTED_LOW (Relays on too long without K1 closed)

else
    K2_and_K3_Coil_State = -1; % Undefined / fallback
end

% if ((K2 == 0 && K3 == 0 && BPCM_Bus_Voltage <= 270) || (K2 == 1 && K3 == 1 && TimeSincePrechargeStart > 90 && BPCM_Bus_Voltage <= 270)) || (K2 == 1 && K3 == 1 && BPCM_Bus_Voltage > 270 && TimeSincePrechargeStart <= 90)
%     K2_and_K3_Coil_State = 2; % NORMAL
% end

end

== matlab function Simulink_Program_June30_K2andK3/Subsystem/Contactor Control/MATLAB Function5 ==
  data: K2 input; K2 output; t input
function K2 = fcn(K2, t)
    if t < 0.25
        if K2 == 1
            K2 = 0;
        end

    elseif  t >= 0.25 && t < 0.34
        if K2 == 0
            K2 = 1;
        end

    elseif t >= 0.34 && t < 0.75 
        if K2 == 0
            K2 = 1;
        end

    else
        if K2 == 1
            K2 = 0;
        end
    end
end

== matlab function Simulink_Program_June30_K2andK3/Subsystem/Contactor Control/MATLAB Function6 ==
  data: K3 input; K3 output; t input
function K3 = fcn(K3, t)
    if t < 0.25
        if K3 == 1
            K3 = 0;
        end

    elseif  t >= 0.25 && t < 0.34
        if K3 == 0
            K3 = 1;
        end

    elseif t >= 0.34 && t < 0.75 
        if K3 == 0 
            K3 = 1;
        end

    else
        if K3 == 1
            K3 = 0;
        end
    end


    % if t >= 0.5 && t < 0.75
    %     if K3 == 1
    %         K3 = 0;
    %     end
    % end
end
